simulink model "gm_uz_pmsm_model_9ph_vnl"  (R2021b)
settings: Solver=FixedStepAuto  StartTime=0.0  StopTime=0.8  RelTol=1e-3
PreLoadFcn:
  | uz_pmsm_model_9ph_init_parameter
undefined symbols (not defined in the file or in its folder): a, b, c, friction_coefficient, inertia, k_i_d, k_i_q, k_p_d, k_p_q, Kpd, L_d, L_o1, L_o2, L_q, L_x1, L_x2, L_y1, L_y2, L_zero, polepair, psi_pm, R_1, static_friction_torque, Tnd, ts
libraries: hdlmdlgenlib x191, hdlsllib x90, dspsigops x19, simulink x17, slpidlib x2, spsAlphaBetaZerotodq0Lib x1, pid_lib x1, spsdq0toAlphaBetaZeroLib x1
(part 3 of 7)

== system gm_uz_pmsm_model_9ph_vnl/Compare/Assert_i_abc1_pl ==
  cosim : Inport
  dut : Inport  Port=2
  AssertEq : Assertion  StopWhenAssertionFail=off
  Compare To Zero : simulink/Logic and Bit Operations/Compare To Zero  relop===  OutDataTypeStr=boolean
  Constant1 : Constant  Value=0  OutDataTypeStr=Inherit: Inherit via back propagation  SampleTime=-1
  Counter : simulink/Sources/Counter Free-Running  NumBits=32  tsamp=-1
  IgnoreCycles : Constant  Value=2  OutDataTypeStr=Inherit: Inherit via back propagation  SampleTime=-1
  Relational Operator : RelationalOperator  Operator=<  OutDataTypeStr=boolean  RndMeth=Nearest
  Relational Operator1 : RelationalOperator  Operator===  OutDataTypeStr=boolean  RndMeth=Nearest
  Switch : Switch  Criteria=u2 ~= 0
  Switch1 : Switch  Criteria=u2 ~= 0
  compare: i_abc1_pl : Scope  NumInputPorts=3
  wires:
  Compare To Zero/1 -> compare: i_abc1_pl/3
  Relational Operator1/1 -> Compare To Zero/1, AssertEq/1  "err"
  Switch1/1 -> compare: i_abc1_pl/1, Relational Operator1/1
  Switch/1 -> compare: i_abc1_pl/2, Relational Operator1/2
  Constant1/1 -> Switch/1, Switch1/1
  Relational Operator/1 -> Switch/2, Switch1/2
  cosim/1 -> Switch1/3  "cosim"
  dut/1 -> Switch/3  "dut ref"
  Counter/1 -> Relational Operator/1
  IgnoreCycles/1 -> Relational Operator/2

== system gm_uz_pmsm_model_9ph_vnl/Compare/Assert_i_abc2_pl ==
  cosim : Inport
  dut : Inport  Port=2
  AssertEq : Assertion  StopWhenAssertionFail=off
  Compare To Zero : simulink/Logic and Bit Operations/Compare To Zero  relop===  OutDataTypeStr=boolean
  Constant1 : Constant  Value=0  OutDataTypeStr=Inherit: Inherit via back propagation  SampleTime=-1
  Counter : simulink/Sources/Counter Free-Running  NumBits=32  tsamp=-1
  IgnoreCycles : Constant  Value=2  OutDataTypeStr=Inherit: Inherit via back propagation  SampleTime=-1
  Relational Operator : RelationalOperator  Operator=<  OutDataTypeStr=boolean  RndMeth=Nearest
  Relational Operator1 : RelationalOperator  Operator===  OutDataTypeStr=boolean  RndMeth=Nearest
  Switch : Switch  Criteria=u2 ~= 0
  Switch1 : Switch  Criteria=u2 ~= 0
  compare: i_abc2_pl : Scope  NumInputPorts=3
  wires:
  Compare To Zero/1 -> compare: i_abc2_pl/3
  Relational Operator1/1 -> Compare To Zero/1, AssertEq/1  "err"
  Switch1/1 -> compare: i_abc2_pl/1, Relational Operator1/1
  Switch/1 -> compare: i_abc2_pl/2, Relational Operator1/2
  Constant1/1 -> Switch/1, Switch1/1
  Relational Operator/1 -> Switch/2, Switch1/2
  cosim/1 -> Switch1/3  "cosim"
  dut/1 -> Switch/3  "dut ref"
  Counter/1 -> Relational Operator/1
  IgnoreCycles/1 -> Relational Operator/2

== system gm_uz_pmsm_model_9ph_vnl/Compare/Assert_i_abc3_pl ==
  cosim : Inport
  dut : Inport  Port=2
  AssertEq : Assertion  StopWhenAssertionFail=off
  Compare To Zero : simulink/Logic and Bit Operations/Compare To Zero  relop===  OutDataTypeStr=boolean
  Constant1 : Constant  Value=0  OutDataTypeStr=Inherit: Inherit via back propagation  SampleTime=-1
  Counter : simulink/Sources/Counter Free-Running  NumBits=32  tsamp=-1
  IgnoreCycles : Constant  Value=2  OutDataTypeStr=Inherit: Inherit via back propagation  SampleTime=-1
  Relational Operator : RelationalOperator  Operator=<  OutDataTypeStr=boolean  RndMeth=Nearest
  Relational Operator1 : RelationalOperator  Operator===  OutDataTypeStr=boolean  RndMeth=Nearest
  Switch : Switch  Criteria=u2 ~= 0
  Switch1 : Switch  Criteria=u2 ~= 0
  compare: i_abc3_pl : Scope  NumInputPorts=3
  wires:
  Compare To Zero/1 -> compare: i_abc3_pl/3
  Relational Operator1/1 -> Compare To Zero/1, AssertEq/1  "err"
  Switch1/1 -> compare: i_abc3_pl/1, Relational Operator1/1
  Switch/1 -> compare: i_abc3_pl/2, Relational Operator1/2
  Constant1/1 -> Switch/1, Switch1/1
  Relational Operator/1 -> Switch/2, Switch1/2
  cosim/1 -> Switch1/3  "cosim"
  dut/1 -> Switch/3  "dut ref"
  Counter/1 -> Relational Operator/1
  IgnoreCycles/1 -> Relational Operator/2

== system gm_uz_pmsm_model_9ph_vnl/Compare/Assert_i_abc_ps ==
  cosim : Inport
  dut : Inport  Port=2
  AssertEq : Assertion  StopWhenAssertionFail=off
  Compare To Zero : simulink/Logic and Bit Operations/Compare To Zero  relop===  OutDataTypeStr=boolean
  Constant1 : Constant  Value=0  OutDataTypeStr=Inherit: Inherit via back propagation  SampleTime=-1
  Counter : simulink/Sources/Counter Free-Running  NumBits=32  tsamp=-1
  IgnoreCycles : Constant  Value=2  OutDataTypeStr=Inherit: Inherit via back propagation  SampleTime=-1
  RelErrCheck : Subsystem
  Relational Operator : RelationalOperator  Operator=<  OutDataTypeStr=boolean  RndMeth=Nearest
  Switch : Switch  Criteria=u2 ~= 0
  Switch1 : Switch  Criteria=u2 ~= 0
  compare: i_abc_ps : Scope  NumInputPorts=3
  wires:
  IgnoreCycles/1 -> Relational Operator/2
  Counter/1 -> Relational Operator/1
  dut/1 -> Switch/3  "dut ref"
  cosim/1 -> Switch1/3  "cosim"
  Relational Operator/1 -> Switch1/2, Switch/2
  Constant1/1 -> Switch1/1, Switch/1
  Switch/1 -> compare: i_abc_ps/2, RelErrCheck/2(In2)
  Switch1/1 -> compare: i_abc_ps/1, RelErrCheck/1(In1)
  RelErrCheck/1(Out1) -> AssertEq/1, Compare To Zero/1  "err"
  Compare To Zero/1 -> compare: i_abc_ps/3

== system gm_uz_pmsm_model_9ph_vnl/Compare/Assert_out_theta_el ==
  cosim : Inport
  dut : Inport  Port=2
  AssertEq : Assertion  StopWhenAssertionFail=off
  Compare To Zero : simulink/Logic and Bit Operations/Compare To Zero  relop===  OutDataTypeStr=boolean
  Constant1 : Constant  Value=0  OutDataTypeStr=Inherit: Inherit via back propagation  SampleTime=-1
  Counter : simulink/Sources/Counter Free-Running  NumBits=32  tsamp=-1
  IgnoreCycles : Constant  Value=2  OutDataTypeStr=Inherit: Inherit via back propagation  SampleTime=-1
  Relational Operator : RelationalOperator  Operator=<  OutDataTypeStr=boolean  RndMeth=Nearest
  Relational Operator1 : RelationalOperator  Operator===  OutDataTypeStr=boolean  RndMeth=Nearest
  Switch : Switch  Criteria=u2 ~= 0
  Switch1 : Switch  Criteria=u2 ~= 0
  compare: out_theta_el : Scope  NumInputPorts=3
  wires:
  Compare To Zero/1 -> compare: out_theta_el/3
  Relational Operator1/1 -> Compare To Zero/1, AssertEq/1  "err"
  Switch1/1 -> compare: out_theta_el/1, Relational Operator1/1
  Switch/1 -> compare: out_theta_el/2, Relational Operator1/2
  Constant1/1 -> Switch/1, Switch1/1
  Relational Operator/1 -> Switch/2, Switch1/2
  cosim/1 -> Switch1/3  "cosim"
  dut/1 -> Switch/3  "dut ref"
  Counter/1 -> Relational Operator/1
  IgnoreCycles/1 -> Relational Operator/2

== system gm_uz_pmsm_model_9ph_vnl/Compare/Assert_outputs ==
  cosim : Inport
  dut : Inport  Port=2
  AssertEq : Assertion  StopWhenAssertionFail=off
  Compare To Zero : simulink/Logic and Bit Operations/Compare To Zero  relop===  OutDataTypeStr=boolean
  Constant1 : Constant  Value=0  OutDataTypeStr=Inherit: Inherit via back propagation  SampleTime=-1
  Counter : simulink/Sources/Counter Free-Running  NumBits=32  tsamp=-1
  IgnoreCycles : Constant  Value=2  OutDataTypeStr=Inherit: Inherit via back propagation  SampleTime=-1
  RelErrCheck : Subsystem
  Relational Operator : RelationalOperator  Operator=<  OutDataTypeStr=boolean  RndMeth=Nearest
  Switch : Switch  Criteria=u2 ~= 0
  Switch1 : Switch  Criteria=u2 ~= 0
  compare: outputs : Scope  NumInputPorts=3
  wires:
  IgnoreCycles/1 -> Relational Operator/2
  Counter/1 -> Relational Operator/1
  dut/1 -> Switch/3  "dut ref"
  cosim/1 -> Switch1/3  "cosim"
  Relational Operator/1 -> Switch1/2, Switch/2
  Constant1/1 -> Switch1/1, Switch/1
  Switch/1 -> compare: outputs/2, RelErrCheck/2(In2)
  Switch1/1 -> compare: outputs/1, RelErrCheck/1(In1)
  RelErrCheck/1(Out1) -> AssertEq/1, Compare To Zero/1  "err"
  Compare To Zero/1 -> compare: outputs/3

== system gm_uz_pmsm_model_9ph_vnl/Compare/CleanupScopes ==

== system gm_uz_pmsm_model_9ph_vnl/Compare/Enable ==

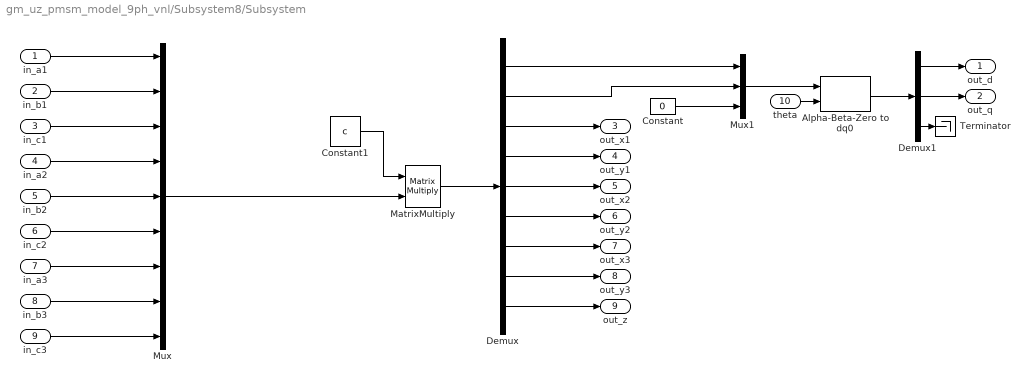
== system gm_uz_pmsm_model_9ph_vnl/Subsystem8/Subsystem ==
  in_a1 : Inport
  in_b1 : Inport  Port=2
  in_c1 : Inport  Port=3
  in_a2 : Inport  Port=4
  in_b2 : Inport  Port=5
  in_c2 : Inport  Port=6
  in_a3 : Inport  Port=7
  in_b3 : Inport  Port=8
  in_c3 : Inport  Port=9
  theta : Inport  Port=10
  Alpha-Beta-Zero to dq0 : spsAlphaBetaZerotodq0Lib/Alpha-Beta-Zero to dq0  Alignment=90 degrees behind phase A axis
      settings: SourceProductBaseCode=PS
  Constant : Constant  Value=0
  Constant1 : Constant  Value=c
  Demux : Demux  Outputs=9
  Demux1 : Demux  Outputs=3
  MatrixMultiply : Product  Multiplication=Matrix(*)
  Mux : Mux  Inputs=9
  Mux1 : Mux  Inputs=3
  Terminator : Terminator
  out_d : Outport
  out_q : Outport  Port=2
  out_x1 : Outport  Port=3
  out_y1 : Outport  Port=4
  out_x2 : Outport  Port=5
  out_y2 : Outport  Port=6
  out_x3 : Outport  Port=7
  out_y3 : Outport  Port=8
  out_z : Outport  Port=9
  wires:
  Demux/6 -> out_y2/1
  Demux/4 -> out_y1/1
  in_a1/1 -> Mux/1
  Demux/5 -> out_x2/1
  MatrixMultiply/1 -> Demux/1
  Demux/3 -> out_x1/1
  in_c3/1 -> Mux/9
  Demux/7 -> out_x3/1
  Demux/8 -> out_y3/1
  Demux/9 -> out_z/1
  theta/1 -> Alpha-Beta-Zero to dq0/2
  Demux1/3 -> Terminator/1
  Demux/1 -> Mux1/1
  Mux1/1 -> Alpha-Beta-Zero to dq0/1
  Demux/2 -> Mux1/2
  Demux1/1 -> out_d/1
  Demux1/2 -> out_q/1
  Constant/1 -> Mux1/3
  Alpha-Beta-Zero to dq0/1 -> Demux1/1
  Constant1/1 -> MatrixMultiply/1
  Mux/1 -> MatrixMultiply/2
  in_b1/1 -> Mux/2
  in_c1/1 -> Mux/3
  in_a2/1 -> Mux/4
  in_b2/1 -> Mux/5
  in_c2/1 -> Mux/6
  in_a3/1 -> Mux/7
  in_b3/1 -> Mux/8

== system gm_uz_pmsm_model_9ph_vnl/Subsystem8/Subsystem11 ==
  setp_Mod_x : Inport
  actual_Mod_x : Inport  Port=2
  Add : Sum  Inputs=+-
  Data Type Conversion8 : DataTypeConversion  OutDataTypeStr=double
  PID Controller2 : pid_lib/PID Controller  Controller=PI  Form=Ideal  TimeDomain=Continuous-time  UseExternalTs=off  SampleTime=-1  IntegratorMethod=Forward Euler  FilterMethod=Forward Euler  ControllerParametersSource=internal  P=Kpd  I=1/Tnd  D=0  UseFilter=on  N=100  TunerSelectOption=Transfer Function Based (PID Tuner App)  InitialConditionSource=internal  InitialConditionForIntegrator=0  InitialConditionForFilter=0  DifferentiatorICPrevScaledInput=0  ExternalReset=none  TrackingMode=off  Kt=1  LimitOutput=on  SatLimitsSource=internal  UpperSaturationLimit=50  LowerSaturationLimit=-50  LinearizeAsGain=on  AntiWindupMode=clamping  Kb=1  POutMin=[]  POutMax=[]  IOutMin=[]  IOutMax=[]  DOutMin=[]  DOutMax=[]  NOutMin=[]  NOutMax=[]  SumOutMin=[]  SumOutMax=[]  SaturationOutMin=[]  SaturationOutMax=[]  PParamMin=[]  PParamMax=[]  IParamMin=[]  IParamMax=[]  DParamMin=[]  DParamMax=[]  NParamMin=[]  NParamMax=[]  KbParamMin=[]  KbParamMax=[]  KtParamMin=[]  KtParamMax=[]  KbOutMin=[]  KbOutMax=[]  KtOutMin=[]  KtOutMax=[]  IntegratorOutMin=[]  IntegratorOutMax=[]  FilterOutMin=[]  FilterOutMax=[]  SumI1OutMin=[]  SumI1OutMax=[]  SumI2OutMin=[]  SumI2OutMax=[]  SumI3OutMin=[]  SumI3OutMax=[]  SumI4OutMin=[]  SumI4OutMax=[]  SumDOutMin=[]  SumDOutMax=[]  DifferentiatorOutMin=[]  DifferentiatorOutMax=[]  FilterDiffOutCoefMin=[]  FilterDiffOutCoefMax=[]  ReciprocalOutMin=[]  ReciprocalOutMax=[]  SumDenOutMin=[]  SumDenOutMax=[]  SumNumOutMin=[]  SumNumOutMax=[]  DivideOutMin=[]  DivideOutMax=[]  UdiffTsProdOutMin=[]  UdiffTsProdOutMax=[]  NTsProdOutMin=[]  NTsProdOutMax=[]  UintegralTsProdOutMin=[]  UintegralTsProdOutMax=[]  UngainTsProdOutMin=[]  UngainTsProdOutMax=[]  IntegratorContinuousStateAttributes=''  IntegratorStateMustResolveToSignalObject=off  IntegratorRTWStateStorageClass=Auto  FilterContinuousStateAttributes=''  FilterStateMustResolveToSignalObject=off  FilterRTWStateStorageClass=Auto  ParallelPVariant=Passthrough  IdealPVariant=InternalParameters  IVariant=InternalParameters  DVariant=Disabled  IntegratorVariant=Continuous  SatVariant=Enabled  AWVariant=ContClampingIdeal  PCopyVariant=InternalParamsIdeal  TRVariant=Disabled  FdbkBlocksVariant=Forward  IdealPFdbkVariant=Disabled  SatFdbkVariant=Disabled  DerivativeFilterVariant=Disabled  NVariant=Disabled  NCopyVariant=Disabled_SignalSpec  FilterICVariant=Disabled  IntegratorICVariant=InternalICs  ExternalResetVariant=Disabled  TRSumVariant=Passthrough  SumFdbkVariant=Disabled  SumVariant=Sum_PI  TsampFilterVariant=InternalTs  TsampNgainVariant=Passthrough  TsampIntegralVariant=Passthrough  ExternalSaturationOutDataTypeStr=Inherit: Same as second input
  out_mod_x : Outport
  wires:
  Add/1 -> Data Type Conversion8/1
  actual_Mod_x/1 -> Add/2
  Data Type Conversion8/1 -> PID Controller2/1
  setp_Mod_x/1 -> Add/1
  PID Controller2/1 -> out_mod_x/1

== system gm_uz_pmsm_model_9ph_vnl/Subsystem8/Subsystem2 ==
  setp_Mod_x : Inport
  actual_Mod_x : Inport  Port=2
  Add : Sum  Inputs=+-
  Data Type Conversion8 : DataTypeConversion  OutDataTypeStr=double
  PID Controller2 : slpidlib/PID Controller  Controller=PI  Form=Ideal  TimeDomain=Continuous-time  UseExternalTs=off  SampleTime=-1  IntegratorMethod=Forward Euler  FilterMethod=Forward Euler  ControllerParametersSource=internal  P=k_p_d  I=k_i_d  D=0  UseFilter=on  N=100  TunerSelectOption=Transfer Function Based (PID Tuner App)  InitialConditionSource=internal  InitialConditionForIntegrator=0  InitialConditionForFilter=0  DifferentiatorICPrevScaledInput=0  ExternalReset=none  TrackingMode=off  Kt=1  LimitOutput=on  SatLimitsSource=internal  UpperSaturationLimit=100  LowerSaturationLimit=-100  LinearizeAsGain=on  AntiWindupMode=clamping  Kb=1  POutMin=[]  POutMax=[]  IOutMin=[]  IOutMax=[]  DOutMin=[]  DOutMax=[]  NOutMin=[]  NOutMax=[]  SumOutMin=[]  SumOutMax=[]  SaturationOutMin=[]  SaturationOutMax=[]  PParamMin=[]  PParamMax=[]  IParamMin=[]  IParamMax=[]  DParamMin=[]  DParamMax=[]  NParamMin=[]  NParamMax=[]  KbParamMin=[]  KbParamMax=[]  KtParamMin=[]  KtParamMax=[]  KbOutMin=[]  KbOutMax=[]  KtOutMin=[]  KtOutMax=[]  IntegratorOutMin=[]  IntegratorOutMax=[]  FilterOutMin=[]  FilterOutMax=[]  SumI1OutMin=[]  SumI1OutMax=[]  SumI2OutMin=[]  SumI2OutMax=[]  SumI3OutMin=[]  SumI3OutMax=[]  SumI4OutMin=[]  SumI4OutMax=[]  SumDOutMin=[]  SumDOutMax=[]  DifferentiatorOutMin=[]  DifferentiatorOutMax=[]  FilterDiffOutCoefMin=[]  FilterDiffOutCoefMax=[]  ReciprocalOutMin=[]  ReciprocalOutMax=[]  SumDenOutMin=[]  SumDenOutMax=[]  SumNumOutMin=[]  SumNumOutMax=[]  DivideOutMin=[]  DivideOutMax=[]  UdiffTsProdOutMin=[]  UdiffTsProdOutMax=[]  NTsProdOutMin=[]  NTsProdOutMax=[]  UintegralTsProdOutMin=[]  UintegralTsProdOutMax=[]  UngainTsProdOutMin=[]  UngainTsProdOutMax=[]  IntegratorContinuousStateAttributes=''  IntegratorStateMustResolveToSignalObject=off  IntegratorRTWStateStorageClass=Auto  FilterContinuousStateAttributes=''  FilterStateMustResolveToSignalObject=off  FilterRTWStateStorageClass=Auto  ParallelPVariant=Passthrough  IdealPVariant=InternalParameters  IVariant=InternalParameters  DVariant=Disabled  IntegratorVariant=Continuous  SatVariant=Enabled  AWVariant=ContClampingIdeal  PCopyVariant=InternalParamsIdeal  TRVariant=Disabled  FdbkBlocksVariant=Forward  IdealPFdbkVariant=Disabled  SatFdbkVariant=Disabled  DerivativeFilterVariant=Disabled  NVariant=Disabled  NCopyVariant=Disabled_SignalSpec  FilterICVariant=Disabled  IntegratorICVariant=InternalICs  ExternalResetVariant=Disabled  TRSumVariant=Passthrough  SumFdbkVariant=Disabled  SumVariant=Sum_PI  TsampFilterVariant=InternalTs  TsampNgainVariant=Passthrough  TsampIntegralVariant=Passthrough  ExternalSaturationOutDataTypeStr=Inherit: Same as second input
  out_mod_x : Outport
  wires:
  Add/1 -> Data Type Conversion8/1
  actual_Mod_x/1 -> Add/2
  Data Type Conversion8/1 -> PID Controller2/1
  setp_Mod_x/1 -> Add/1
  PID Controller2/1 -> out_mod_x/1

== system gm_uz_pmsm_model_9ph_vnl/Subsystem8/Subsystem3 ==
  setp_Mod_x : Inport
  actual_Mod_x : Inport  Port=2
  Add : Sum  Inputs=+-
  Data Type Conversion8 : DataTypeConversion  OutDataTypeStr=double
  PID Controller2 : slpidlib/PID Controller  Controller=PI  Form=Ideal  TimeDomain=Continuous-time  UseExternalTs=off  SampleTime=-1  IntegratorMethod=Forward Euler  FilterMethod=Forward Euler  ControllerParametersSource=internal  P=k_p_q  I=k_i_q  D=0  UseFilter=on  N=100  TunerSelectOption=Transfer Function Based (PID Tuner App)  InitialConditionSource=internal  InitialConditionForIntegrator=0  InitialConditionForFilter=0  DifferentiatorICPrevScaledInput=0  ExternalReset=none  TrackingMode=off  Kt=1  LimitOutput=on  SatLimitsSource=internal  UpperSaturationLimit=100  LowerSaturationLimit=-100  LinearizeAsGain=on  AntiWindupMode=clamping  Kb=1  POutMin=[]  POutMax=[]  IOutMin=[]  IOutMax=[]  DOutMin=[]  DOutMax=[]  NOutMin=[]  NOutMax=[]  SumOutMin=[]  SumOutMax=[]  SaturationOutMin=[]  SaturationOutMax=[]  PParamMin=[]  PParamMax=[]  IParamMin=[]  IParamMax=[]  DParamMin=[]  DParamMax=[]  NParamMin=[]  NParamMax=[]  KbParamMin=[]  KbParamMax=[]  KtParamMin=[]  KtParamMax=[]  KbOutMin=[]  KbOutMax=[]  KtOutMin=[]  KtOutMax=[]  IntegratorOutMin=[]  IntegratorOutMax=[]  FilterOutMin=[]  FilterOutMax=[]  SumI1OutMin=[]  SumI1OutMax=[]  SumI2OutMin=[]  SumI2OutMax=[]  SumI3OutMin=[]  SumI3OutMax=[]  SumI4OutMin=[]  SumI4OutMax=[]  SumDOutMin=[]  SumDOutMax=[]  DifferentiatorOutMin=[]  DifferentiatorOutMax=[]  FilterDiffOutCoefMin=[]  FilterDiffOutCoefMax=[]  ReciprocalOutMin=[]  ReciprocalOutMax=[]  SumDenOutMin=[]  SumDenOutMax=[]  SumNumOutMin=[]  SumNumOutMax=[]  DivideOutMin=[]  DivideOutMax=[]  UdiffTsProdOutMin=[]  UdiffTsProdOutMax=[]  NTsProdOutMin=[]  NTsProdOutMax=[]  UintegralTsProdOutMin=[]  UintegralTsProdOutMax=[]  UngainTsProdOutMin=[]  UngainTsProdOutMax=[]  IntegratorContinuousStateAttributes=''  IntegratorStateMustResolveToSignalObject=off  IntegratorRTWStateStorageClass=Auto  FilterContinuousStateAttributes=''  FilterStateMustResolveToSignalObject=off  FilterRTWStateStorageClass=Auto  ParallelPVariant=Passthrough  IdealPVariant=InternalParameters  IVariant=InternalParameters  DVariant=Disabled  IntegratorVariant=Continuous  SatVariant=Enabled  AWVariant=ContClampingIdeal  PCopyVariant=InternalParamsIdeal  TRVariant=Disabled  FdbkBlocksVariant=Forward  IdealPFdbkVariant=Disabled  SatFdbkVariant=Disabled  DerivativeFilterVariant=Disabled  NVariant=Disabled  NCopyVariant=Disabled_SignalSpec  FilterICVariant=Disabled  IntegratorICVariant=InternalICs  ExternalResetVariant=Disabled  TRSumVariant=Passthrough  SumFdbkVariant=Disabled  SumVariant=Sum_PI  TsampFilterVariant=InternalTs  TsampNgainVariant=Passthrough  TsampIntegralVariant=Passthrough  ExternalSaturationOutDataTypeStr=Inherit: Same as second input
  out_mod_x : Outport
  wires:
  PID Controller2/1 -> out_mod_x/1
  setp_Mod_x/1 -> Add/1
  Data Type Conversion8/1 -> PID Controller2/1
  actual_Mod_x/1 -> Add/2
  Add/1 -> Data Type Conversion8/1

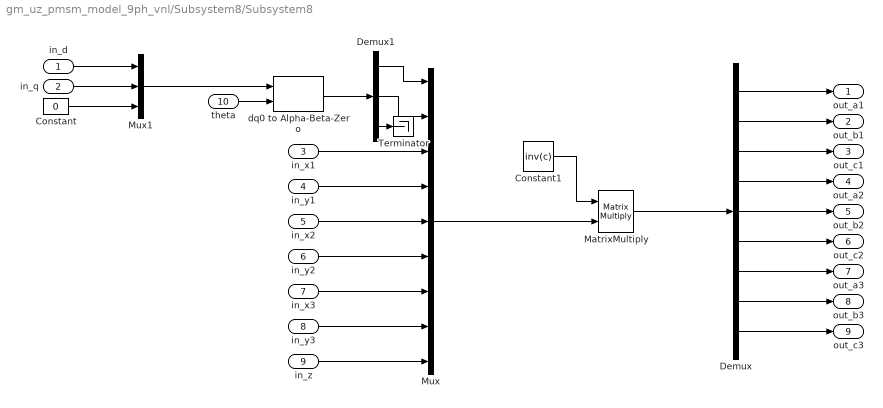
== system gm_uz_pmsm_model_9ph_vnl/Subsystem8/Subsystem8 ==
  in_d : Inport
  in_q : Inport  Port=2
  in_x1 : Inport  Port=3
  in_y1 : Inport  Port=4
  in_x2 : Inport  Port=5
  in_y2 : Inport  Port=6
  in_x3 : Inport  Port=7
  in_y3 : Inport  Port=8
  in_z : Inport  Port=9
  theta : Inport  Port=10
  Constant : Constant  Value=0
  Constant1 : Constant  Value=inv(c)
  Demux : Demux  Outputs=9
  Demux1 : Demux  Outputs=3
  MatrixMultiply : Product  Multiplication=Matrix(*)
  Mux : Mux  Inputs=9
  Mux1 : Mux  Inputs=3
  Terminator : Terminator
  dq0 to Alpha-Beta-Zero : spsdq0toAlphaBetaZeroLib/dq0 to Alpha-Beta-Zero  Alignment=90 degrees behind phase A axis
      settings: SourceProductBaseCode=PS
  out_a1 : Outport
  out_b1 : Outport  Port=2
  out_c1 : Outport  Port=3
  out_a2 : Outport  Port=4
  out_b2 : Outport  Port=5
  out_c2 : Outport  Port=6
  out_a3 : Outport  Port=7
  out_b3 : Outport  Port=8
  out_c3 : Outport  Port=9
  wires:
  in_x3/1 -> Mux/7
  in_y3/1 -> Mux/8
  MatrixMultiply/1 -> Demux/1
  in_y2/1 -> Mux/6
  Demux/1 -> out_a1/1
  in_x1/1 -> Mux/3
  in_y1/1 -> Mux/4
  Mux/1 -> MatrixMultiply/2
  in_x2/1 -> Mux/5
  in_z/1 -> Mux/9
  Constant/1 -> Mux1/3
  in_q/1 -> Mux1/2
  in_d/1 -> Mux1/1
  Mux1/1 -> dq0 to Alpha-Beta-Zero/1
  theta/1 -> dq0 to Alpha-Beta-Zero/2
  dq0 to Alpha-Beta-Zero/1 -> Demux1/1
  Demux1/1 -> Mux/1
  Demux1/2 -> Mux/2
  Demux1/3 -> Terminator/1
  Constant1/1 -> MatrixMultiply/1
  Demux/2 -> out_b1/1
  Demux/3 -> out_c1/1
  Demux/4 -> out_a2/1
  Demux/6 -> out_c2/1
  Demux/5 -> out_b2/1
  Demux/8 -> out_b3/1
  Demux/9 -> out_c3/1
  Demux/7 -> out_a3/1

== system gm_uz_pmsm_model_9ph_vnl/uz_pmsm_model_9ph/Add ==
  In1 : Inport
  In2 : Inport  Port=2
  Add : Sum  Inputs=+-  OutDataTypeStr=single  SampleTime=1e-08
  Add_pd1 : Delay  DelayLength=6
  Out1 : Outport
  wires:
  Add_pd1/1 -> Out1/1
  Add/1 -> Add_pd1/1
  In2/1 -> Add/2
  In1/1 -> Add/1

== system gm_uz_pmsm_model_9ph_vnl/uz_pmsm_model_9ph/Add1 ==
  In1 : Inport
  In2 : Inport  Port=2
  Add1 : Sum  Inputs=+-  OutDataTypeStr=single  SampleTime=1e-08
  Add1_pd1 : Delay  DelayLength=6
  Out1 : Outport
  wires:
  Add1_pd1/1 -> Out1/1
  Add1/1 -> Add1_pd1/1
  In2/1 -> Add1/2
  In1/1 -> Add1/1

== system gm_uz_pmsm_model_9ph_vnl/uz_pmsm_model_9ph/Add2 ==
  In1 : Inport
  In2 : Inport  Port=2
  Add2 : Sum  Inputs=+-  OutDataTypeStr=single  SampleTime=1e-08
  Add2_pd1 : Delay  DelayLength=6
  Out1 : Outport
  wires:
  Add2_pd1/1 -> Out1/1
  Add2/1 -> Add2_pd1/1
  In2/1 -> Add2/2
  In1/1 -> Add2/1

== system gm_uz_pmsm_model_9ph_vnl/uz_pmsm_model_9ph/Add3 ==
  In1 : Inport
  In2 : Inport  Port=2
  Add3 : Sum  Inputs=+-  OutDataTypeStr=single  SampleTime=1e-08
  Add3_pd1 : Delay  DelayLength=6
  Out1 : Outport
  wires:
  Add3_pd1/1 -> Out1/1
  Add3/1 -> Add3_pd1/1
  In2/1 -> Add3/2
  In1/1 -> Add3/1

== system gm_uz_pmsm_model_9ph_vnl/uz_pmsm_model_9ph/Add4 ==
  In1 : Inport
  In2 : Inport  Port=2
  Add4 : Sum  Inputs=+-  OutDataTypeStr=single  SampleTime=1e-08
  Add4_pd1 : Delay  DelayLength=6
  Out1 : Outport
  wires:
  Add4_pd1/1 -> Out1/1
  Add4/1 -> Add4_pd1/1
  In2/1 -> Add4/2
  In1/1 -> Add4/1

== system gm_uz_pmsm_model_9ph_vnl/uz_pmsm_model_9ph/Add5 ==
  In1 : Inport
  In2 : Inport  Port=2
  Add5 : Sum  Inputs=+-  OutDataTypeStr=single  SampleTime=1e-08
  Add5_pd1 : Delay  DelayLength=6
  Out1 : Outport
  wires:
  Add5_pd1/1 -> Out1/1
  Add5/1 -> Add5_pd1/1
  In2/1 -> Add5/2
  In1/1 -> Add5/1

== system gm_uz_pmsm_model_9ph_vnl/uz_pmsm_model_9ph/Add6 ==
  In1 : Inport
  In2 : Inport  Port=2
  Add6 : Sum  Inputs=+-  OutDataTypeStr=single  SampleTime=1e-08
  Add6_pd1 : Delay  DelayLength=6
  Out1 : Outport
  wires:
  Add6_pd1/1 -> Out1/1
  Add6/1 -> Add6_pd1/1
  In2/1 -> Add6/2
  In1/1 -> Add6/1

== system gm_uz_pmsm_model_9ph_vnl/uz_pmsm_model_9ph/Cast To Double ==
  In1 : Inport
  Cast To Double : DataTypeConversion  OutDataTypeStr=single  SampleTime=1e-08
  Cast To Double_pd1 : Delay  DelayLength=6
  Out1 : Outport
  wires:
  Cast To Double_pd1/1 -> Out1/1
  Cast To Double/1 -> Cast To Double_pd1/1
  In1/1 -> Cast To Double/1

== system gm_uz_pmsm_model_9ph_vnl/uz_pmsm_model_9ph/Cast To Double1 ==
  In1 : Inport
  Cast To Double1 : DataTypeConversion  OutDataTypeStr=single  SampleTime=1e-08
  Cast To Double1_pd1 : Delay  DelayLength=6
  Out1 : Outport
  wires:
  Cast To Double1_pd1/1 -> Out1/1
  Cast To Double1/1 -> Cast To Double1_pd1/1
  In1/1 -> Cast To Double1/1

== system gm_uz_pmsm_model_9ph_vnl/uz_pmsm_model_9ph/Cast To Double2 ==
  In1 : Inport
  Cast To Double2 : DataTypeConversion  OutDataTypeStr=single  SampleTime=1e-08
  Cast To Double2_pd1 : Delay  DelayLength=6
  Out1 : Outport
  wires:
  Cast To Double2_pd1/1 -> Out1/1
  Cast To Double2/1 -> Cast To Double2_pd1/1
  In1/1 -> Cast To Double2/1

== system gm_uz_pmsm_model_9ph_vnl/uz_pmsm_model_9ph/Data Type Conversion1 ==
  In1 : Inport
  Data Type Conversion1 : DataTypeConversion  OutDataTypeStr=fixdt(1, 25, 12)  RndMeth=Nearest  SampleTime=1e-08
  Data Type Conversion1_pd1 : Delay  DelayLength=6
  Out1 : Outport
  wires:
  Data Type Conversion1_pd1/1 -> Out1/1
  Data Type Conversion1/1 -> Data Type Conversion1_pd1/1
  In1/1 -> Data Type Conversion1/1

== system gm_uz_pmsm_model_9ph_vnl/uz_pmsm_model_9ph/Data Type Conversion11 ==
  In1 : Inport
  Data Type Conversion11 : DataTypeConversion  OutDataTypeStr=double  RndMeth=Nearest  SampleTime=1e-08
  Data Type Conversion11_pd1 : Delay  DelayLength=3
  Out1 : Outport
  wires:
  Data Type Conversion11_pd1/1 -> Out1/1
  Data Type Conversion11/1 -> Data Type Conversion11_pd1/1
  In1/1 -> Data Type Conversion11/1

== system gm_uz_pmsm_model_9ph_vnl/uz_pmsm_model_9ph/Data Type Conversion12 ==
  In1 : Inport
  Data Type Conversion12 : DataTypeConversion  OutDataTypeStr=double  RndMeth=Nearest  SampleTime=1e-08
  Data Type Conversion12_pd1 : Delay  DelayLength=3
  Out1 : Outport
  wires:
  Data Type Conversion12_pd1/1 -> Out1/1
  Data Type Conversion12/1 -> Data Type Conversion12_pd1/1
  In1/1 -> Data Type Conversion12/1

== system gm_uz_pmsm_model_9ph_vnl/uz_pmsm_model_9ph/Data Type Conversion13 ==
  In1 : Inport
  Data Type Conversion13 : DataTypeConversion  OutDataTypeStr=single  RndMeth=Nearest  SampleTime=1e-08
  Data Type Conversion13_pd1 : Delay  DelayLength=3
  Out1 : Outport
  wires:
  Data Type Conversion13_pd1/1 -> Out1/1
  Data Type Conversion13/1 -> Data Type Conversion13_pd1/1
  In1/1 -> Data Type Conversion13/1

== system gm_uz_pmsm_model_9ph_vnl/uz_pmsm_model_9ph/Data Type Conversion14 ==
  In1 : Inport
  Data Type Conversion14 : DataTypeConversion  OutDataTypeStr=double  RndMeth=Nearest  SampleTime=1e-08
  Data Type Conversion14_pd1 : Delay  DelayLength=3
  Out1 : Outport
  wires:
  Data Type Conversion14_pd1/1 -> Out1/1
  Data Type Conversion14/1 -> Data Type Conversion14_pd1/1
  In1/1 -> Data Type Conversion14/1

== system gm_uz_pmsm_model_9ph_vnl/uz_pmsm_model_9ph/Data Type Conversion141 ==
  In1 : Inport
  Data Type Conversion141 : DataTypeConversion  OutDataTypeStr=single  RndMeth=Nearest  SampleTime=1e-08
  Data Type Conversion141_pd1 : Delay  DelayLength=3
  Out1 : Outport
  wires:
  Data Type Conversion141_pd1/1 -> Out1/1
  Data Type Conversion141/1 -> Data Type Conversion141_pd1/1
  In1/1 -> Data Type Conversion141/1

== system gm_uz_pmsm_model_9ph_vnl/uz_pmsm_model_9ph/Data Type Conversion15 ==
  In1 : Inport
  Data Type Conversion15 : DataTypeConversion  OutDataTypeStr=single  RndMeth=Nearest  SampleTime=1e-08
  Data Type Conversion15_pd1 : Delay  DelayLength=3
  Out1 : Outport
  wires:
  Data Type Conversion15_pd1/1 -> Out1/1
  Data Type Conversion15/1 -> Data Type Conversion15_pd1/1
  In1/1 -> Data Type Conversion15/1

== system gm_uz_pmsm_model_9ph_vnl/uz_pmsm_model_9ph/Data Type Conversion16 ==
  In1 : Inport
  Data Type Conversion16 : DataTypeConversion  OutDataTypeStr=single  RndMeth=Nearest  SampleTime=1e-08
  Data Type Conversion16_pd1 : Delay  DelayLength=3
  Out1 : Outport
  wires:
  Data Type Conversion16_pd1/1 -> Out1/1
  Data Type Conversion16/1 -> Data Type Conversion16_pd1/1
  In1/1 -> Data Type Conversion16/1

== system gm_uz_pmsm_model_9ph_vnl/uz_pmsm_model_9ph/Data Type Conversion17 ==
  In1 : Inport
  Data Type Conversion17 : DataTypeConversion  OutDataTypeStr=single  RndMeth=Nearest  SampleTime=1e-08
  Data Type Conversion17_pd1 : Delay  DelayLength=3
  Out1 : Outport
  wires:
  Data Type Conversion17_pd1/1 -> Out1/1
  Data Type Conversion17/1 -> Data Type Conversion17_pd1/1
  In1/1 -> Data Type Conversion17/1

== system gm_uz_pmsm_model_9ph_vnl/uz_pmsm_model_9ph/Data Type Conversion18 ==
  In1 : Inport
  Data Type Conversion18 : DataTypeConversion  OutDataTypeStr=single  RndMeth=Nearest  SampleTime=1e-08
  Data Type Conversion18_pd1 : Delay  DelayLength=3
  Out1 : Outport
  wires:
  Data Type Conversion18_pd1/1 -> Out1/1
  Data Type Conversion18/1 -> Data Type Conversion18_pd1/1
  In1/1 -> Data Type Conversion18/1

== system gm_uz_pmsm_model_9ph_vnl/uz_pmsm_model_9ph/Data Type Conversion19 ==
  In1 : Inport
  Data Type Conversion19 : DataTypeConversion  OutDataTypeStr=single  RndMeth=Nearest  SampleTime=1e-08
  Data Type Conversion19_pd1 : Delay  DelayLength=3
  Out1 : Outport
  wires:
  Data Type Conversion19_pd1/1 -> Out1/1
  Data Type Conversion19/1 -> Data Type Conversion19_pd1/1
  In1/1 -> Data Type Conversion19/1

== system gm_uz_pmsm_model_9ph_vnl/uz_pmsm_model_9ph/Data Type Conversion20 ==
  In1 : Inport
  Data Type Conversion20 : DataTypeConversion  OutDataTypeStr=single  RndMeth=Nearest  SampleTime=1e-08
  Data Type Conversion20_pd1 : Delay  DelayLength=3
  Out1 : Outport
  wires:
  Data Type Conversion20_pd1/1 -> Out1/1
  Data Type Conversion20/1 -> Data Type Conversion20_pd1/1
  In1/1 -> Data Type Conversion20/1

== system gm_uz_pmsm_model_9ph_vnl/uz_pmsm_model_9ph/Data Type Conversion21 ==
  In1 : Inport
  Data Type Conversion21 : DataTypeConversion  OutDataTypeStr=double  RndMeth=Nearest  SampleTime=1e-08
  Data Type Conversion21_pd1 : Delay  DelayLength=3
  Out1 : Outport
  wires:
  Data Type Conversion21_pd1/1 -> Out1/1
  Data Type Conversion21/1 -> Data Type Conversion21_pd1/1
  In1/1 -> Data Type Conversion21/1

== system gm_uz_pmsm_model_9ph_vnl/uz_pmsm_model_9ph/Data Type Conversion22 ==
  In1 : Inport
  Data Type Conversion22 : DataTypeConversion  OutDataTypeStr=double  RndMeth=Nearest  SampleTime=1e-08
  Data Type Conversion22_pd1 : Delay  DelayLength=3
  Out1 : Outport
  wires:
  Data Type Conversion22_pd1/1 -> Out1/1
  Data Type Conversion22/1 -> Data Type Conversion22_pd1/1
  In1/1 -> Data Type Conversion22/1

== system gm_uz_pmsm_model_9ph_vnl/uz_pmsm_model_9ph/Data Type Conversion23 ==
  In1 : Inport
  Data Type Conversion23 : DataTypeConversion  OutDataTypeStr=single  RndMeth=Nearest  SampleTime=1e-08
  Data Type Conversion23_pd1 : Delay  DelayLength=3
  Out1 : Outport
  wires:
  Data Type Conversion23_pd1/1 -> Out1/1
  Data Type Conversion23/1 -> Data Type Conversion23_pd1/1
  In1/1 -> Data Type Conversion23/1

== system gm_uz_pmsm_model_9ph_vnl/uz_pmsm_model_9ph/Data Type Conversion24 ==
  In1 : Inport
  Data Type Conversion24 : DataTypeConversion  OutDataTypeStr=double  RndMeth=Nearest  SampleTime=1e-08
  Data Type Conversion24_pd1 : Delay  DelayLength=3
  Out1 : Outport
  wires:
  Data Type Conversion24_pd1/1 -> Out1/1
  Data Type Conversion24/1 -> Data Type Conversion24_pd1/1
  In1/1 -> Data Type Conversion24/1

== system gm_uz_pmsm_model_9ph_vnl/uz_pmsm_model_9ph/Data Type Conversion25 ==
  In1 : Inport
  Data Type Conversion25 : DataTypeConversion  OutDataTypeStr=double  RndMeth=Nearest  SampleTime=1e-08
  Data Type Conversion25_pd1 : Delay  DelayLength=3
  Out1 : Outport
  wires:
  Data Type Conversion25_pd1/1 -> Out1/1
  Data Type Conversion25/1 -> Data Type Conversion25_pd1/1
  In1/1 -> Data Type Conversion25/1

== system gm_uz_pmsm_model_9ph_vnl/uz_pmsm_model_9ph/Data Type Conversion26 ==
  In1 : Inport
  Data Type Conversion26 : DataTypeConversion  OutDataTypeStr=double  RndMeth=Nearest  SampleTime=1e-08
  Data Type Conversion26_pd1 : Delay  DelayLength=3
  Out1 : Outport
  wires:
  Data Type Conversion26_pd1/1 -> Out1/1
  Data Type Conversion26/1 -> Data Type Conversion26_pd1/1
  In1/1 -> Data Type Conversion26/1

== system gm_uz_pmsm_model_9ph_vnl/uz_pmsm_model_9ph/Data Type Conversion27 ==
  In1 : Inport
  Data Type Conversion27 : DataTypeConversion  OutDataTypeStr=double  RndMeth=Nearest  SampleTime=1e-08
  Data Type Conversion27_pd1 : Delay  DelayLength=3
  Out1 : Outport
  wires:
  Data Type Conversion27_pd1/1 -> Out1/1
  Data Type Conversion27/1 -> Data Type Conversion27_pd1/1
  In1/1 -> Data Type Conversion27/1

== system gm_uz_pmsm_model_9ph_vnl/uz_pmsm_model_9ph/Data Type Conversion28 ==
  In1 : Inport
  Data Type Conversion28 : DataTypeConversion  OutDataTypeStr=double  RndMeth=Nearest  SampleTime=1e-08
  Data Type Conversion28_pd1 : Delay  DelayLength=3
  Out1 : Outport
  wires:
  Data Type Conversion28_pd1/1 -> Out1/1
  Data Type Conversion28/1 -> Data Type Conversion28_pd1/1
  In1/1 -> Data Type Conversion28/1

== system gm_uz_pmsm_model_9ph_vnl/uz_pmsm_model_9ph/Data Type Conversion29 ==
  In1 : Inport
  Data Type Conversion29 : DataTypeConversion  OutDataTypeStr=double  RndMeth=Nearest  SampleTime=1e-08
  Data Type Conversion29_pd1 : Delay  DelayLength=3
  Out1 : Outport
  wires:
  Data Type Conversion29_pd1/1 -> Out1/1
  Data Type Conversion29/1 -> Data Type Conversion29_pd1/1
  In1/1 -> Data Type Conversion29/1

== system gm_uz_pmsm_model_9ph_vnl/uz_pmsm_model_9ph/Data Type Conversion3 ==
  In1 : Inport
  Data Type Conversion3 : DataTypeConversion  OutDataTypeStr=double  RndMeth=Nearest  SampleTime=1e-08
  Data Type Conversion3_pd1 : Delay  DelayLength=3
  Out1 : Outport
  wires:
  Data Type Conversion3_pd1/1 -> Out1/1
  Data Type Conversion3/1 -> Data Type Conversion3_pd1/1
  In1/1 -> Data Type Conversion3/1

== system gm_uz_pmsm_model_9ph_vnl/uz_pmsm_model_9ph/Data Type Conversion30 ==
  In1 : Inport
  Data Type Conversion30 : DataTypeConversion  OutDataTypeStr=double  RndMeth=Nearest  SampleTime=1e-08
  Data Type Conversion30_pd1 : Delay  DelayLength=3
  Out1 : Outport
  wires:
  Data Type Conversion30_pd1/1 -> Out1/1
  Data Type Conversion30/1 -> Data Type Conversion30_pd1/1
  In1/1 -> Data Type Conversion30/1

== system gm_uz_pmsm_model_9ph_vnl/uz_pmsm_model_9ph/Data Type Conversion31 ==
  In1 : Inport
  Data Type Conversion31 : DataTypeConversion  OutDataTypeStr=single  RndMeth=Nearest  SampleTime=1e-08
  Data Type Conversion31_pd1 : Delay  DelayLength=3
  Out1 : Outport
  wires:
  Data Type Conversion31_pd1/1 -> Out1/1
  Data Type Conversion31/1 -> Data Type Conversion31_pd1/1
  In1/1 -> Data Type Conversion31/1

== system gm_uz_pmsm_model_9ph_vnl/uz_pmsm_model_9ph/Data Type Conversion32 ==
  In1 : Inport
  Data Type Conversion32 : DataTypeConversion  OutDataTypeStr=single  RndMeth=Nearest  SampleTime=1e-08
  Data Type Conversion32_pd1 : Delay  DelayLength=3
  Out1 : Outport
  wires:
  Data Type Conversion32_pd1/1 -> Out1/1
  Data Type Conversion32/1 -> Data Type Conversion32_pd1/1
  In1/1 -> Data Type Conversion32/1

== system gm_uz_pmsm_model_9ph_vnl/uz_pmsm_model_9ph/Data Type Conversion33 ==
  In1 : Inport
  Data Type Conversion33 : DataTypeConversion  OutDataTypeStr=double  RndMeth=Nearest  SampleTime=1e-08
  Data Type Conversion33_pd1 : Delay  DelayLength=3
  Out1 : Outport
  wires:
  Data Type Conversion33_pd1/1 -> Out1/1
  Data Type Conversion33/1 -> Data Type Conversion33_pd1/1
  In1/1 -> Data Type Conversion33/1

== system gm_uz_pmsm_model_9ph_vnl/uz_pmsm_model_9ph/Data Type Conversion331 ==
  In1 : Inport
  Data Type Conversion331 : DataTypeConversion  OutDataTypeStr=double  RndMeth=Nearest  SampleTime=1e-08
  Data Type Conversion331_pd1 : Delay  DelayLength=3
  Out1 : Outport
  wires:
  Data Type Conversion331_pd1/1 -> Out1/1
  Data Type Conversion331/1 -> Data Type Conversion331_pd1/1
  In1/1 -> Data Type Conversion331/1

== system gm_uz_pmsm_model_9ph_vnl/uz_pmsm_model_9ph/Data Type Conversion37 ==
  In1 : Inport
  Data Type Conversion37 : DataTypeConversion  OutDataTypeStr=single  RndMeth=Nearest  SampleTime=1e-08
  Data Type Conversion37_pd1 : Delay  DelayLength=6
  Out1 : Outport
  wires:
  Data Type Conversion37_pd1/1 -> Out1/1
  Data Type Conversion37/1 -> Data Type Conversion37_pd1/1
  In1/1 -> Data Type Conversion37/1

== system gm_uz_pmsm_model_9ph_vnl/uz_pmsm_model_9ph/Data Type Conversion5 ==
  In1 : Inport
  Data Type Conversion5 : DataTypeConversion  OutDataTypeStr=double  RndMeth=Nearest  SampleTime=1e-08
  Data Type Conversion5_pd1 : Delay  DelayLength=3
  Out1 : Outport
  wires:
  Data Type Conversion5_pd1/1 -> Out1/1
  Data Type Conversion5/1 -> Data Type Conversion5_pd1/1
  In1/1 -> Data Type Conversion5/1

== system gm_uz_pmsm_model_9ph_vnl/uz_pmsm_model_9ph/Data Type Conversion51 ==
  In1 : Inport
  Data Type Conversion51 : DataTypeConversion  OutDataTypeStr=single  RndMeth=Nearest  SampleTime=1e-08
  Data Type Conversion51_pd1 : Delay  DelayLength=6
  Out1 : Outport
  wires:
  Data Type Conversion51_pd1/1 -> Out1/1
  Data Type Conversion51/1 -> Data Type Conversion51_pd1/1
  In1/1 -> Data Type Conversion51/1

== system gm_uz_pmsm_model_9ph_vnl/uz_pmsm_model_9ph/Data Type Conversion81 ==
  In1 : Inport
  Data Type Conversion81 : DataTypeConversion  OutDataTypeStr=single  RndMeth=Nearest  SampleTime=1e-08
  Data Type Conversion81_pd1 : Delay  DelayLength=3
  Out1 : Outport
  wires:
  Data Type Conversion81_pd1/1 -> Out1/1
  Data Type Conversion81/1 -> Data Type Conversion81_pd1/1
  In1/1 -> Data Type Conversion81/1

== system gm_uz_pmsm_model_9ph_vnl/uz_pmsm_model_9ph/Data Type Conversion9 ==
  In1 : Inport
  Data Type Conversion9 : DataTypeConversion  OutDataTypeStr=fixdt(1, 25, 12)  RndMeth=Nearest  SampleTime=1e-08
  Data Type Conversion9_pd1 : Delay  DelayLength=6
  Out1 : Outport
  wires:
  Data Type Conversion9_pd1/1 -> Out1/1
  Data Type Conversion9/1 -> Data Type Conversion9_pd1/1
  In1/1 -> Data Type Conversion9/1

== system gm_uz_pmsm_model_9ph_vnl/uz_pmsm_model_9ph/Divide ==
  In1 : Inport
  In2 : Inport  Port=2
  Divide : Product  Inputs=**  OutDataTypeStr=single  SampleTime=1e-08
  Divide_pd1 : Delay  DelayLength=6
  Out1 : Outport
  wires:
  Divide_pd1/1 -> Out1/1
  Divide/1 -> Divide_pd1/1
  In2/1 -> Divide/2
  In1/1 -> Divide/1

== system gm_uz_pmsm_model_9ph_vnl/uz_pmsm_model_9ph/Divide1 ==
  In1 : Inport
  In2 : Inport  Port=2
  Divide1 : Product  Inputs=**  OutDataTypeStr=single  SampleTime=1e-08
  Divide1_pd1 : Delay  DelayLength=6
  Out1 : Outport
  wires:
  Divide1_pd1/1 -> Out1/1
  Divide1/1 -> Divide1_pd1/1
  In2/1 -> Divide1/2
  In1/1 -> Divide1/1

== system gm_uz_pmsm_model_9ph_vnl/uz_pmsm_model_9ph/Divide10 ==
  In1 : Inport
  In2 : Inport  Port=2
  Divide10 : Product  Inputs=**  OutDataTypeStr=single  SampleTime=1e-08
  Divide10_pd1 : Delay  DelayLength=6
  Out1 : Outport
  wires:
  Divide10_pd1/1 -> Out1/1
  Divide10/1 -> Divide10_pd1/1
  In2/1 -> Divide10/2
  In1/1 -> Divide10/1

== system gm_uz_pmsm_model_9ph_vnl/uz_pmsm_model_9ph/Divide11 ==
  In1 : Inport
  In2 : Inport  Port=2
  Divide11 : Product  Inputs=**  OutDataTypeStr=single  SampleTime=1e-08
  Divide11_pd1 : Delay  DelayLength=6
  Out1 : Outport
  wires:
  Divide11_pd1/1 -> Out1/1
  Divide11/1 -> Divide11_pd1/1
  In2/1 -> Divide11/2
  In1/1 -> Divide11/1

== system gm_uz_pmsm_model_9ph_vnl/uz_pmsm_model_9ph/Divide12 ==
  In1 : Inport
  In2 : Inport  Port=2
  Divide12 : Product  Inputs=**  OutDataTypeStr=single  SampleTime=1e-08
  Divide12_pd1 : Delay  DelayLength=6
  Out1 : Outport
  wires:
  Divide12_pd1/1 -> Out1/1
  Divide12/1 -> Divide12_pd1/1
  In2/1 -> Divide12/2
  In1/1 -> Divide12/1

== system gm_uz_pmsm_model_9ph_vnl/uz_pmsm_model_9ph/Divide13 ==
  In1 : Inport
  In2 : Inport  Port=2
  Divide13 : Product  Inputs=**  OutDataTypeStr=single  SampleTime=1e-08
  Divide13_pd1 : Delay  DelayLength=6
  Out1 : Outport
  wires:
  Divide13_pd1/1 -> Out1/1
  Divide13/1 -> Divide13_pd1/1
  In2/1 -> Divide13/2
  In1/1 -> Divide13/1

== system gm_uz_pmsm_model_9ph_vnl/uz_pmsm_model_9ph/Divide2 ==
  In1 : Inport
  In2 : Inport  Port=2
  Divide2 : Product  Inputs=**  OutDataTypeStr=single  SampleTime=1e-08
  Divide2_pd1 : Delay  DelayLength=6
  Out1 : Outport
  wires:
  Divide2_pd1/1 -> Out1/1
  Divide2/1 -> Divide2_pd1/1
  In2/1 -> Divide2/2
  In1/1 -> Divide2/1

== system gm_uz_pmsm_model_9ph_vnl/uz_pmsm_model_9ph/Divide3 ==
  In1 : Inport
  In2 : Inport  Port=2
  Divide3 : Product  Inputs=**  OutDataTypeStr=single  SampleTime=1e-08
  Divide3_pd1 : Delay  DelayLength=6
  Out1 : Outport
  wires:
  Divide3_pd1/1 -> Out1/1
  Divide3/1 -> Divide3_pd1/1
  In2/1 -> Divide3/2
  In1/1 -> Divide3/1

== system gm_uz_pmsm_model_9ph_vnl/uz_pmsm_model_9ph/Divide4 ==
  In1 : Inport
  In2 : Inport  Port=2
  Divide4 : Product  Inputs=**  OutDataTypeStr=single  SampleTime=1e-08
  Divide4_pd1 : Delay  DelayLength=6
  Out1 : Outport
  wires:
  Divide4_pd1/1 -> Out1/1
  Divide4/1 -> Divide4_pd1/1
  In2/1 -> Divide4/2
  In1/1 -> Divide4/1

== system gm_uz_pmsm_model_9ph_vnl/uz_pmsm_model_9ph/Divide5 ==
  In1 : Inport
  In2 : Inport  Port=2
  Divide5 : Product  Inputs=**  OutDataTypeStr=single  SampleTime=1e-08
  Divide5_pd1 : Delay  DelayLength=6
  Out1 : Outport
  wires:
  Divide5_pd1/1 -> Out1/1
  Divide5/1 -> Divide5_pd1/1
  In2/1 -> Divide5/2
  In1/1 -> Divide5/1

== system gm_uz_pmsm_model_9ph_vnl/uz_pmsm_model_9ph/Divide6 ==
  In1 : Inport
  In2 : Inport  Port=2
  Divide6 : Product  Inputs=**  OutDataTypeStr=single  SampleTime=1e-08
  Divide6_pd1 : Delay  DelayLength=6
  Out1 : Outport
  wires:
  Divide6_pd1/1 -> Out1/1
  Divide6/1 -> Divide6_pd1/1
  In2/1 -> Divide6/2
  In1/1 -> Divide6/1

== system gm_uz_pmsm_model_9ph_vnl/uz_pmsm_model_9ph/Divide7 ==
  In1 : Inport
  In2 : Inport  Port=2
  Divide7 : Product  Inputs=**  OutDataTypeStr=single  SampleTime=1e-08
  Divide7_pd1 : Delay  DelayLength=6
  Out1 : Outport
  wires:
  Divide7_pd1/1 -> Out1/1
  Divide7/1 -> Divide7_pd1/1
  In2/1 -> Divide7/2
  In1/1 -> Divide7/1

== system gm_uz_pmsm_model_9ph_vnl/uz_pmsm_model_9ph/Divide8 ==
  In1 : Inport
  In2 : Inport  Port=2
  Divide8 : Product  Inputs=**  OutDataTypeStr=single  SampleTime=1e-08
  Divide8_pd1 : Delay  DelayLength=6
  Out1 : Outport
  wires:
  Divide8_pd1/1 -> Out1/1
  Divide8/1 -> Divide8_pd1/1
  In2/1 -> Divide8/2
  In1/1 -> Divide8/1

== system gm_uz_pmsm_model_9ph_vnl/uz_pmsm_model_9ph/Divide9 ==
  In1 : Inport
  In2 : Inport  Port=2
  Divide9 : Product  Inputs=**  OutDataTypeStr=single  SampleTime=1e-08
  Divide9_pd1 : Delay  DelayLength=6
  Out1 : Outport
  wires:
  Divide9_pd1/1 -> Out1/1
  Divide9/1 -> Divide9_pd1/1
  In2/1 -> Divide9/2
  In1/1 -> Divide9/1

== system gm_uz_pmsm_model_9ph_vnl/uz_pmsm_model_9ph/Factor ==
  In1 : Inport
  In2 : Inport  Port=2
  Factor : Product  Inputs=**  OutDataTypeStr=single  SampleTime=1e-08
  Factor_pd1 : Delay  DelayLength=6
  Out1 : Outport
  wires:
  Factor_pd1/1 -> Out1/1
  Factor/1 -> Factor_pd1/1
  In2/1 -> Factor/2
  In1/1 -> Factor/1

== system gm_uz_pmsm_model_9ph_vnl/uz_pmsm_model_9ph/Gain ==
  In1 : Inport
  In2 : Inport  Port=2
  Gain : Product  Inputs=**  OutDataTypeStr=double  SampleTime=1e-08
  Gain_pd1 : Delay  DelayLength=6
  Out1 : Outport
  wires:
  Gain_pd1/1 -> Out1/1
  Gain/1 -> Gain_pd1/1
  In2/1 -> Gain/2
  In1/1 -> Gain/1

== system gm_uz_pmsm_model_9ph_vnl/uz_pmsm_model_9ph/Gain1 ==
  In1 : Inport
  In2 : Inport  Port=2
  Gain1 : Product  Inputs=**  OutDataTypeStr=double  SampleTime=1e-08
  Gain1_pd1 : Delay  DelayLength=6
  Out1 : Outport
  wires:
  Gain1_pd1/1 -> Out1/1
  Gain1/1 -> Gain1_pd1/1
  In2/1 -> Gain1/2
  In1/1 -> Gain1/1

== system gm_uz_pmsm_model_9ph_vnl/uz_pmsm_model_9ph/Gain2 ==
  In1 : Inport
  In2 : Inport  Port=2
  Gain2 : Product  Inputs=**  OutDataTypeStr=double  SampleTime=1e-08
  Gain2_pd1 : Delay  DelayLength=6
  Out1 : Outport
  wires:
  Gain2_pd1/1 -> Out1/1
  Gain2/1 -> Gain2_pd1/1
  In2/1 -> Gain2/2
  In1/1 -> Gain2/1

== system gm_uz_pmsm_model_9ph_vnl/uz_pmsm_model_9ph/Gain3 ==
  In1 : Inport
  In2 : Inport  Port=2
  Gain3 : Product  Inputs=**  OutDataTypeStr=double  SampleTime=1e-08
  Gain3_pd1 : Delay  DelayLength=6
  Out1 : Outport
  wires:
  Gain3_pd1/1 -> Out1/1
  Gain3/1 -> Gain3_pd1/1
  In2/1 -> Gain3/2
  In1/1 -> Gain3/1

== system gm_uz_pmsm_model_9ph_vnl/uz_pmsm_model_9ph/Gain4 ==
  In1 : Inport
  In2 : Inport  Port=2
  Gain4 : Product  Inputs=**  OutDataTypeStr=double  SampleTime=1e-08
  Gain4_pd1 : Delay  DelayLength=6
  Out1 : Outport
  wires:
  Gain4_pd1/1 -> Out1/1
  Gain4/1 -> Gain4_pd1/1
  In2/1 -> Gain4/2
  In1/1 -> Gain4/1

== system gm_uz_pmsm_model_9ph_vnl/uz_pmsm_model_9ph/Gain5 ==
  In1 : Inport
  In2 : Inport  Port=2
  Gain5 : Product  Inputs=**  OutDataTypeStr=double  SampleTime=1e-08
  Gain5_pd1 : Delay  DelayLength=6
  Out1 : Outport
  wires:
  Gain5_pd1/1 -> Out1/1
  Gain5/1 -> Gain5_pd1/1
  In2/1 -> Gain5/2
  In1/1 -> Gain5/1

== system gm_uz_pmsm_model_9ph_vnl/uz_pmsm_model_9ph/Gain6 ==
  In1 : Inport
  In2 : Inport  Port=2
  Gain6 : Product  Inputs=**  OutDataTypeStr=double  SampleTime=1e-08
  Gain6_pd1 : Delay  DelayLength=6
  Out1 : Outport
  wires:
  Gain6_pd1/1 -> Out1/1
  Gain6/1 -> Gain6_pd1/1
  In2/1 -> Gain6/2
  In1/1 -> Gain6/1

== system gm_uz_pmsm_model_9ph_vnl/uz_pmsm_model_9ph/Gain7 ==
  In1 : Inport
  In2 : Inport  Port=2
  Gain7 : Product  Inputs=**  OutDataTypeStr=double  SampleTime=1e-08
  Gain7_pd1 : Delay  DelayLength=6
  Out1 : Outport
  wires:
  Gain7_pd1/1 -> Out1/1
  Gain7/1 -> Gain7_pd1/1
  In2/1 -> Gain7/2
  In1/1 -> Gain7/1

== system gm_uz_pmsm_model_9ph_vnl/uz_pmsm_model_9ph/Gain8 ==
  In1 : Inport
  In2 : Inport  Port=2
  Gain8 : Product  Inputs=**  OutDataTypeStr=double  SampleTime=1e-08
  Gain8_pd1 : Delay  DelayLength=6
  Out1 : Outport
  wires:
  Gain8_pd1/1 -> Out1/1
  Gain8/1 -> Gain8_pd1/1
  In2/1 -> Gain8/2
  In1/1 -> Gain8/1

== system gm_uz_pmsm_model_9ph_vnl/uz_pmsm_model_9ph/Gain9 ==
  In1 : Inport
  In2 : Inport  Port=2
  Gain9 : Product  Inputs=**  OutDataTypeStr=double  SampleTime=1e-08
  Gain9_pd1 : Delay  DelayLength=6
  Out1 : Outport
  wires:
  Gain9_pd1/1 -> Out1/1
  Gain9/1 -> Gain9_pd1/1
  In2/1 -> Gain9/2
  In1/1 -> Gain9/1

== system gm_uz_pmsm_model_9ph_vnl/uz_pmsm_model_9ph/Line-Line to Phase voltage ==
  In1 : Inport  OutDataTypeStr=single  PortDimensions=[3]  SampleTime=1e-08
  Complex to Real-Imag : ComplexToRealImag  SampleTime=1e-08
  Constant : Constant  Value=single(0)  OutDataTypeStr=single  SampleTime=1e-08
  Constant1 : Constant  Value=complex(0.5, -0.28867512941360474)  OutDataTypeStr=single  SampleTime=1e-08
  Product : Subsystem
      mask Display: disp('NFP\nmul');
  Product1 : Subsystem
      mask Display: disp('NFP\nmul');
  Product2 : Subsystem
      mask Display: disp('NFP\nmul');
  Product3 : Subsystem
      mask Display: disp('NFP\nmul');
  Product_AC_minus_BD : Subsystem
      mask Display: disp('NFP\nadd');
  Product_AD_plus_BC : Subsystem
      mask Display: disp('NFP\nadd');
  Product_C2ReIm_1 : ComplexToRealImag  SampleTime=1e-08
  Product_C2ReIm_2 : ComplexToRealImag  SampleTime=1e-08
  Product_ReIm2Complex : RealImagToComplex  SampleTime=1e-08
  Real-Imag to Complex : RealImagToComplex  ConstantPart=single(0)  SampleTime=1e-08
  abc   to   alpha_beta_0 : Subsystem
  abc   to   alpha_beta_0_out1_2_term2 : Terminator
  alpha_beta_0   to   abc : Subsystem
  delayMatch{,1..3} (4 alike) : Delay  DelayLength=double(24)  InitialCondition=0  SampleTime=1e-08
  mux : Mux  Inputs=3
  t : Demux  Outputs=3
  Out1 : Outport  SampleTime=1e-08
  wires:
  In1/1 -> abc   to   alpha_beta_0/1("a, b, c")
  Product_AD_plus_BC/1(Out1) -> Product_ReIm2Complex/2
  Product_AC_minus_BD/1(Out1) -> Product_ReIm2Complex/1
  Product3/1(Out1) -> Product_AD_plus_BC/2(In2)
  Product2/1(Out1) -> Product_AC_minus_BD/2(In2)
  Product1/1(Out1) -> Product_AD_plus_BC/1(In1)
  Product/1(Out1) -> Product_AC_minus_BD/1(In1)
  Product_C2ReIm_2/1 -> delayMatch/1, delayMatch3/1
  Product_C2ReIm_2/2 -> delayMatch1/1, delayMatch2/1
  delayMatch2/1 -> Product2/2(In2)
  delayMatch3/1 -> Product3/2(In2)
  delayMatch1/1 -> Product1/2(In2)
  delayMatch/1 -> Product/2(In2)
  Product_C2ReIm_1/2 -> Product2/1(In1), Product3/1(In1)
  Product_C2ReIm_1/1 -> Product/1(In1), Product1/1(In1)
  t/3 -> abc   to   alpha_beta_0_out1_2_term2/1
  t/2 -> Real-Imag to Complex/2
  t/1 -> Real-Imag to Complex/1
  alpha_beta_0   to   abc/1("a, b, c") -> Out1/1
  abc   to   alpha_beta_0/1("alpha, beta, 0 ") -> t/1
  Real-Imag to Complex/1 -> Product_C2ReIm_1/1
  Product_ReIm2Complex/1 -> Complex to Real-Imag/1
  mux/1 -> alpha_beta_0   to   abc/1("alpha, beta, 0  ")
  Constant1/1 -> Product_C2ReIm_2/1
  Constant/1 -> mux/3
  Complex to Real-Imag/2 -> mux/2
  Complex to Real-Imag/1 -> mux/1
